simulink model "eje3_3_3_modelo"  (R2019b)
settings: Solver=ode15s  StartTime=0.0  StopTime=500  RelTol=1e-3  AbsTol=0.001
values from neighbouring files (symbols this model uses):
  C = 1    [ejercicio3_3_1.m]
  L = 1    [ejercicio3_3_1.m]
  R = 100    [ejercicio3_3_1.m]
settings Model: Creator=Fer  LastModifiedBy=Fer
settings SolverCC: AutoScaleAbsTol=off

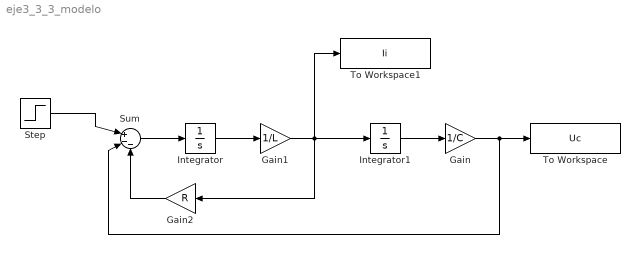
== system eje3_3_3_modelo ==
  Gain : Gain  Gain=1/C
  Gain1 : Gain  Gain=1/L
  Gain2 : Gain  Gain=R
  Integrator : Integrator
  Integrator1 : Integrator
  Step : Step  Time=0  SampleTime=0
  Sum : Sum  Inputs=|+--
  To Workspace : ToWorkspace  VariableName=Uc  SampleTime=-1
  To Workspace1 : ToWorkspace  VariableName=Ii  SampleTime=-1
  wires:
  Step/1 -> Sum/1
  Sum/1 -> Integrator/1
  Integrator/1 -> Gain1/1
  Gain2/1 -> Sum/3
  Gain1/1 -> To Workspace1/1, Integrator1/1, Gain2/1
  Integrator1/1 -> Gain/1
  Gain/1 -> To Workspace/1, Sum/2
